simulink model "Traffic_Light"  (R2020b)
settings: Solver=FixedStepDiscrete  StartTime=0.0  StopTime=150  FixedStep=0.1  RelTol=1e-3  EnableMultiTasking=on
undefined symbols (not defined in the file): DiscIntNeverNeededParam
libraries: simulink x1
settings Model: Creator=Shivashis  LastModifiedBy=Shivashis
settings DataIOCC: SaveFormat=Array

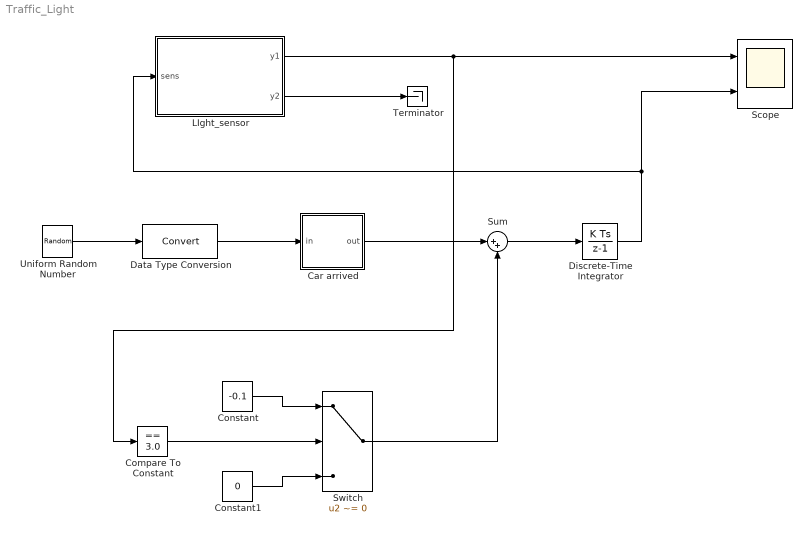
== system Traffic_Light ==
  Car arrived : Stateflow chart  TreatAsAtomicUnit=on
  Compare To Constant : simulink/Logic and Bit Operations/Compare To Constant  relop===  const=3.0  OutDataTypeStr=boolean
  Constant : Constant  Value=-0.1
  Constant1 : Constant  Value=0
  Data Type Conversion : DataTypeConversion
  Discrete-Time Integrator : DiscreteIntegrator  SampleTime=-1  ICPrevOutput=DiscIntNeverNeededParam  ICPrevScaledInput=DiscIntNeverNeededParam
  LIght_sensor : Stateflow chart  TreatAsAtomicUnit=on
  Scope : Scope  NumInputPorts=2
  Sum : Sum  Inputs=|++
  Switch : Switch  Criteria=u2 ~= 0
  Terminator : Terminator
  Uniform Random Number : UniformRandomNumber  Minimum=0  Maximum=100  Seed=177836  SampleTime=0
  wires:
  Uniform Random Number/1 -> Data Type Conversion/1
  Data Type Conversion/1 -> Car arrived/1(in)
  Car arrived/1(out) -> Sum/1
  Sum/1 -> Discrete-Time Integrator/1
  Compare To Constant/1 -> Switch/2
  Constant/1 -> Switch/1
  Constant1/1 -> Switch/3
  Switch/1 -> Sum/2
  Discrete-Time Integrator/1 -> Scope/2, LIght_sensor/1(sens)
  LIght_sensor/1(y1) -> Compare To Constant/1, Scope/1
  LIght_sensor/2(y2) -> Terminator/1

== stateflow chart Traffic_Light/LIght_sensor ==
  settings: stateMachineType=MOORE_MACHINE  initializeOutput=1
  state Stop
    y1=RED;
    y2=GREEN;
  state Stop_for_Traffic
    y1=RED;
    y2=GREEN;
  state Stop_to_Go
    y1=RED;
    y2=YELLOW;
  state Go_to_Stop
    y1=YELLOW
    y2=RED;
  state Go
    y1=GREEN;
    y2=RED;
  (default) -> Stop
  Stop -> Stop_for_Traffic : after(20,tick)
  Stop_for_Traffic -> Stop_to_Go : [sens]
  Go_to_Stop -> Stop : after(3,tick)
  Stop_to_Go -> Go : after(3,tick)
  Go -> Go_to_Stop : after(10,tick)
  data: sens input double; y1 output double; y2 output double; RED constant uint8 =1; GREEN constant double =2; YELLOW constant double =3

== stateflow chart Traffic_Light/Car arrived ==
  (default) -> (junction 1) : {out=in>98;}
  data: in input int8; out output double
